simulink model "sl_subsys_fcncall11"  (Simulink 7.6)
settings: Solver=FixedStepDiscrete  StartTime=0.0  StopTime=30  RelTol=1e-3
settings Model: Creator=The MathWorks Inc.
settings DataIOCC: SaveFormat=StructureWithTime
settings OptimizationCC: BlockReduction=off
settings DebuggingCC: UnderspecifiedInitializationDetection=Simplified  StrictBusMsg=ErrorOnBusTreatedAsVector
settings SFSimCC: SimParseCustomCode=off

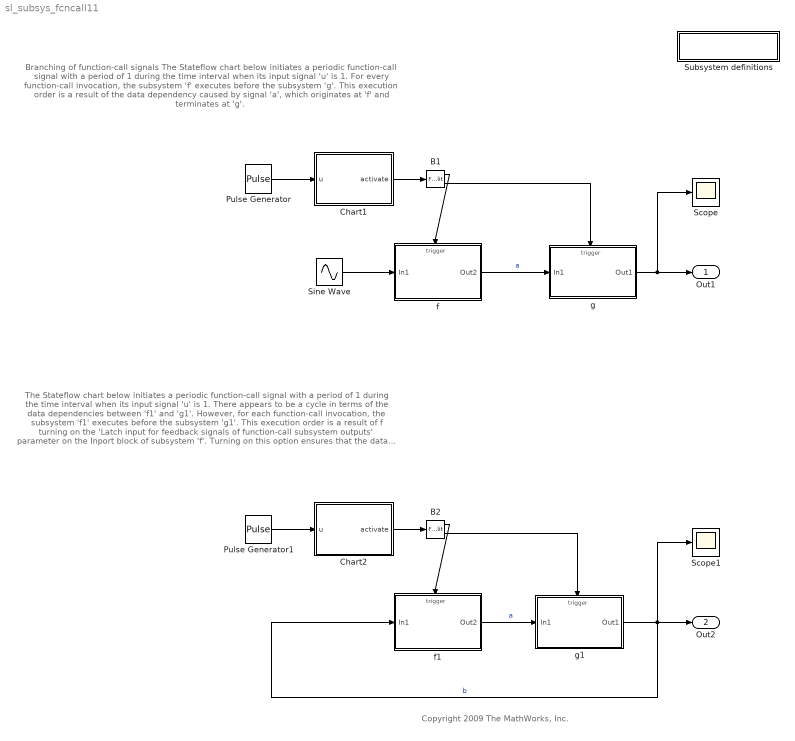
== system sl_subsys_fcncall11 ==
  note: Branching of function-call signals
      |
      | The Stateflow chart below initiates a periodic function-call signal with a period of 1
      | during the time interval when its input signal 'u' is 1. For every function-call
      | invocation, the subsystem 'f' executes before the subsystem 'g'. This execution
      | order is a result of the data dependency caused by signal  'a', which originates
      | at 'f' and terminates at 'g'.
  note: The Stateflow chart below initiates a periodic function-call signal with a period of 1 during the
      | time interval when its input signal 'u' is 1. There appears to be a cycle in terms of the data
      | dependencies between 'f1' and 'g1'. However, for each function-call invocation, the subsystem
      | 'f1' executes before the subsystem 'g1'. This execution order is a result of f turning on the
      | 'Latch input for feedback signals of function-call subsystem outputs' parameter on the Inport
      | block of subsystem 'f'. Turning on this option ensures that the data dependency caused by
      | signal 'b' is ignored. Consequently, subsystem 'f1' uses the 'g1' output computed at the
      | previous time step.
      |
      | Note that setting the 'Latch input for feedback signals of function-call subsystem outputs'
      | to 'Off' in the Inport block of subsystem 'f1' results in a data-dependency violation error.
  note: Copyright 2009 The MathWorks, Inc.
  " Subsystem definitions" : Subsystem
      settings: OpenFcn=helpview([matlabroot,'/toolbox/simulink/simdemos/simfeatures/html/sl_subsys_definitions.html']);
      mask Display: disp('Subsystem\ndefinitions')
  B1 : FunctionCallSplit
  B2 : FunctionCallSplit
  Chart1 : Stateflow chart  TreatAsAtomicUnit=on
  Chart2 : Stateflow chart  TreatAsAtomicUnit=on
  Pulse Generator : DiscretePulseGenerator  Period=10  PulseWidth=5
  Pulse Generator1 : DiscretePulseGenerator  Period=10  PulseWidth=5
  Scope : Scope
  Scope1 : Scope
  Sine Wave : Sin  SampleTime=1
  f : Subsystem  TreatAsAtomicUnit=on
  f1 : Subsystem  TreatAsAtomicUnit=on
  g : Subsystem  TreatAsAtomicUnit=on
  g1 : Subsystem  TreatAsAtomicUnit=on
  Out1 : Outport
  Out2 : Outport  Port=2
  wires:
  g/1(Out1) -> Out1/1, Scope/1
  Chart1/1(activate) -> B1/1
  B1/1 -> f/Trigger
  B1/2 -> g/Trigger
  f/1(Out2) -> g/1(In1)  "a"
  Sine Wave/1 -> f/1(In1)
  Pulse Generator/1 -> Chart1/1(u)
  g1/1(Out1) -> Scope1/1, Out2/1, f1/1(In1)  "b"
  Chart2/1(activate) -> B2/1
  B2/1 -> f1/Trigger
  B2/2 -> g1/Trigger
  f1/1(Out2) -> g1/1(In1)  "a"
  Pulse Generator1/1 -> Chart2/1(u)

== system sl_subsys_fcncall11/ Subsystem definitions ==

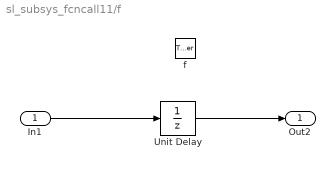
== system sl_subsys_fcncall11/f ==
  In1 : Inport
  f : TriggerPort  TriggerType=function-call  SampleTimeType=periodic
  Unit Delay : UnitDelay  SampleTime=-1
      settings: AttributesFormatString=IC: %<X0>
  Out2 : Outport  OutputWhenDisabled=reset  InitialOutput=0
  wires:
  In1/1 -> Unit Delay/1
  Unit Delay/1 -> Out2/1

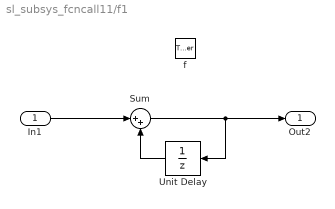
== system sl_subsys_fcncall11/f1 ==
  In1 : Inport
      settings: LatchInputForFeedbackSignals=on
  f : TriggerPort  TriggerType=function-call  SampleTimeType=periodic
  Sum : Sum  Inputs=|++
  Unit Delay : UnitDelay  X0=1  SampleTime=-1
      settings: AttributesFormatString=IC: %<X0>
  Out2 : Outport  OutputWhenDisabled=reset  InitialOutput=1
  wires:
  Sum/1 -> Out2/1, Unit Delay/1
  In1/1 -> Sum/1
  Unit Delay/1 -> Sum/2

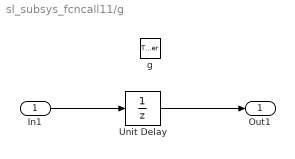
== system sl_subsys_fcncall11/g ==
  In1 : Inport
  g : TriggerPort  TriggerType=function-call  SampleTimeType=periodic
      settings: AttributesFormatString=%<StatesWhenEnabling>
  Unit Delay : UnitDelay  SampleTime=-1
      settings: AttributesFormatString=IC: %<X0>
  Out1 : Outport  OutputWhenDisabled=reset  InitialOutput=0
  wires:
  Unit Delay/1 -> Out1/1
  In1/1 -> Unit Delay/1

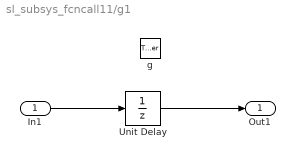
== system sl_subsys_fcncall11/g1 ==
  In1 : Inport
  g : TriggerPort  TriggerType=function-call  SampleTimeType=periodic
      settings: AttributesFormatString=%<StatesWhenEnabling>
  Unit Delay : UnitDelay  X0=1  SampleTime=-1
      settings: AttributesFormatString=IC: %<X0>
  Out1 : Outport  OutputWhenDisabled=reset  InitialOutput=1
  wires:
  In1/1 -> Unit Delay/1
  Unit Delay/1 -> Out1/1

== stateflow chart Chart2 ==
  state OFF
  state ON/
    entry:activate;
    bind: activate;
  OFF -> ON : [u == 1]
  ON -> OFF [order 1] : [u == 0]
  (default) -> OFF
  ON -> ON [order 2]
  data: u input double
  events: activate output FUNCTION_CALL_EVENT

== stateflow chart Chart1 ==
  state OFF
  state ON/
    entry:activate;
    bind: activate;
  OFF -> ON : [u == 1]
  ON -> OFF [order 1] : [u == 0]
  (default) -> OFF
  ON -> ON [order 2]
  data: u input double
  events: activate output FUNCTION_CALL_EVENT
